simulink model "hnn_without_bias_3_neurons"  (R2024b)
settings: Solver=VariableStepAuto  StartTime=0.0  StopTime=10.0  RelTol=1e-3
settings Model: Creator=merlin  LastModifiedBy=merlin

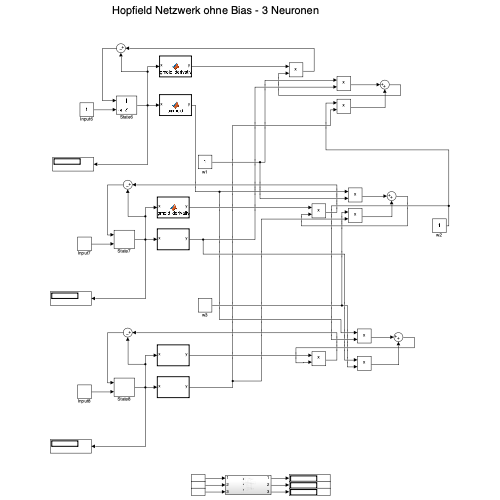
[thumbnail: Simulink's stored preview of the top-level diagram]
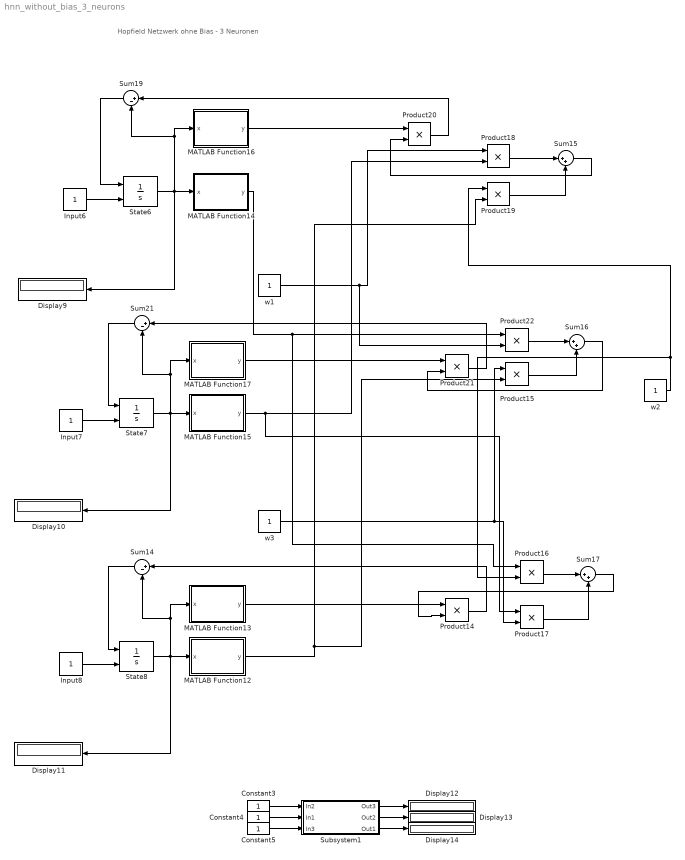
== system hnn_without_bias_3_neurons ==
  note: Hopfield Netzwerk ohne Bias - 3 Neuronen
  Constant3 : Constant
  Constant4 : Constant
  Constant5 : Constant
  Display{9..14} (6 alike) : Display
  Input6 : Constant
  Input7 : Constant
  Input8 : Constant
  MATLAB Function12 : MATLAB Function  TreatAsAtomicUnit=on
  MATLAB Function13 : MATLAB Function  TreatAsAtomicUnit=on
  MATLAB Function14 : MATLAB Function  TreatAsAtomicUnit=on
  MATLAB Function15 : MATLAB Function  TreatAsAtomicUnit=on
  MATLAB Function16 : MATLAB Function  TreatAsAtomicUnit=on
  MATLAB Function17 : MATLAB Function  TreatAsAtomicUnit=on
  Product{14..22} (9 alike) : Product
  State6 : Integrator  InitialConditionSource=external
  State7 : Integrator  InitialConditionSource=external
  State8 : Integrator  InitialConditionSource=external
  Subsystem1 : Subsystem
  Sum14 : Sum  Inputs=|+-
  Sum15 : Sum  Inputs=|++
  Sum16 : Sum  Inputs=|++
  Sum17 : Sum  Inputs=|++
  Sum19 : Sum  Inputs=|+-
  Sum21 : Sum  Inputs=|+-
  w1 : Constant
  w2 : Constant
  w3 : Constant
  wires:
  Sum14/1 -> State8/1
  Sum21/1 -> State7/1
  Sum17/1 -> Product14/2
  Product22/1 -> Sum16/1
  Input7/1 -> State7/2
  State7/1 -> Display10/1, Sum21/2, MATLAB Function17/1(x), MATLAB Function15/1(x)
  Product20/1 -> Sum19/1
  w3/1 -> Product17/2, Product15/1
  MATLAB Function16/1(y) -> Product20/1
  State6/1 -> Display9/1, Sum19/2, MATLAB Function16/1(x), MATLAB Function14/1(x)
  MATLAB Function12/1(y) -> Product15/2, Product19/2
  Subsystem1/2(Out2) -> Display13/1
  w2/1 -> Product16/2, Product19/1
  MATLAB Function17/1(y) -> Product21/1
  Input8/1 -> State8/2
  Sum19/1 -> State6/1
  Constant5/1 -> Subsystem1/3(In3)
  Constant4/1 -> Subsystem1/2(In1)
  Product15/1 -> Sum16/2
  MATLAB Function15/1(y) -> Product17/1, Product18/2
  Product14/1 -> Sum14/1
  Subsystem1/1(Out3) -> Display12/1
  Input6/1 -> State6/2
  State8/1 -> Display11/1, Sum14/2, MATLAB Function13/1(x), MATLAB Function12/1(x)
  w1/1 -> Product22/2, Product18/1
  Constant3/1 -> Subsystem1/1(In2)
  MATLAB Function14/1(y) -> Product16/1, Product22/1
  Product19/1 -> Sum15/2
  Product17/1 -> Sum17/2
  Sum15/1 -> Product20/2
  Product16/1 -> Sum17/1
  Product18/1 -> Sum15/1
  MATLAB Function13/1(y) -> Product14/1
  Sum16/1 -> Product21/2
  Subsystem1/3(Out1) -> Display14/1
  Product21/1 -> Sum21/1

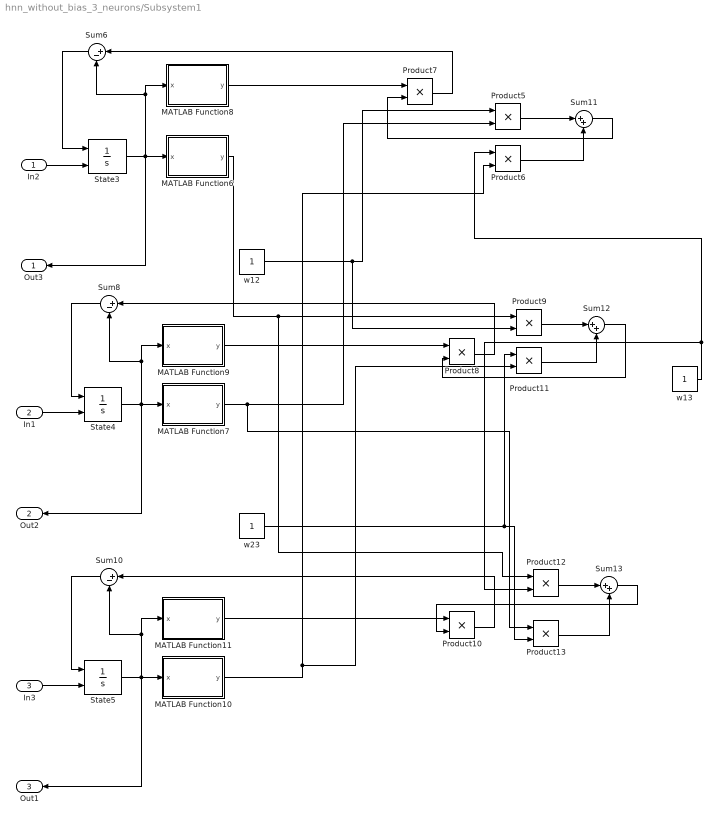
== system hnn_without_bias_3_neurons/Subsystem1 ==
  In2 : Inport
  In1 : Inport  Port=2
  In3 : Inport  Port=3
  MATLAB Function10 : MATLAB Function  TreatAsAtomicUnit=on
  MATLAB Function11 : MATLAB Function  TreatAsAtomicUnit=on
  MATLAB Function6 : MATLAB Function  TreatAsAtomicUnit=on
  MATLAB Function7 : MATLAB Function  TreatAsAtomicUnit=on
  MATLAB Function8 : MATLAB Function  TreatAsAtomicUnit=on
  MATLAB Function9 : MATLAB Function  TreatAsAtomicUnit=on
  Product{5..13} (9 alike) : Product
  State3 : Integrator  InitialConditionSource=external
  State4 : Integrator  InitialConditionSource=external
  State5 : Integrator  InitialConditionSource=external
  Sum10 : Sum  Inputs=|+-
  Sum11 : Sum  Inputs=|++
  Sum12 : Sum  Inputs=|++
  Sum13 : Sum  Inputs=|++
  Sum6 : Sum  Inputs=|+-
  Sum8 : Sum  Inputs=|+-
  w12 : Constant
  w13 : Constant
  w23 : Constant
  Out3 : Outport
  Out2 : Outport  Port=2
  Out1 : Outport  Port=3
  wires:
  Product9/1 -> Sum12/1
  Product13/1 -> Sum13/2
  Sum11/1 -> Product7/2
  Sum10/1 -> State5/1
  MATLAB Function7/1(y) -> Product13/1, Product5/2
  MATLAB Function9/1(y) -> Product8/1
  Product5/1 -> Sum11/1
  w12/1 -> Product9/2, Product5/1
  State5/1 -> Out1/1, Sum10/2, MATLAB Function11/1(x), MATLAB Function10/1(x)
  MATLAB Function8/1(y) -> Product7/1
  MATLAB Function11/1(y) -> Product10/1
  Sum13/1 -> Product10/2
  MATLAB Function6/1(y) -> Product12/1, Product9/1
  Product12/1 -> Sum13/1
  MATLAB Function10/1(y) -> Product11/2, Product6/2
  State4/1 -> Out2/1, Sum8/2, MATLAB Function9/1(x), MATLAB Function7/1(x)
  Sum8/1 -> State4/1
  Product8/1 -> Sum8/1
  State3/1 -> Out3/1, Sum6/2, MATLAB Function8/1(x), MATLAB Function6/1(x)
  Sum6/1 -> State3/1
  Product7/1 -> Sum6/1
  Product6/1 -> Sum11/2
  In1/1 -> State4/2
  Sum12/1 -> Product8/2
  In3/1 -> State5/2
  w23/1 -> Product13/2, Product11/1
  Product11/1 -> Sum12/2
  Product10/1 -> Sum10/1
  w13/1 -> Product12/2, Product6/1
  In2/1 -> State3/2

== matlab function hnn_without_bias_3_neurons/MATLAB Function13 ==
  data: x input; y output
function y = sigmoid_derivative(x)
sigmoid = 1 ./ (1 + exp(-x));
y = sigmoid .* (1 - sigmoid);
end

== matlab function hnn_without_bias_3_neurons/MATLAB Function14 ==
  data: x input; y output
function y = sigmoid(x)
y = 1 ./ (1 + exp(-x));
end

== matlab function hnn_without_bias_3_neurons/MATLAB Function15 ==
  data: x input; y output
function y = sigmoid(x)
y = 1 ./ (1 + exp(-x));
end

== matlab function hnn_without_bias_3_neurons/MATLAB Function16 ==
  data: x input; y output
function y = sigmoid_derivative(x)
sigmoid = 1 ./ (1 + exp(-x));
y = sigmoid .* (1 - sigmoid);
end

== matlab function hnn_without_bias_3_neurons/MATLAB Function17 ==
  data: x input; y output
function y = sigmoid_derivative(x)
sigmoid = 1 ./ (1 + exp(-x));
y = sigmoid .* (1 - sigmoid);
end

== matlab function hnn_without_bias_3_neurons/Subsystem1/MATLAB Function10 ==
  data: x input; y output
function y = sigmoid(x)
y = 1 ./ (1 + exp(-x));
end

== matlab function hnn_without_bias_3_neurons/Subsystem1/MATLAB Function11 ==
  data: x input; y output
function y = sigmoid_derivative(x)
sigmoid = 1 ./ (1 + exp(-x));
y = sigmoid .* (1 - sigmoid);
end

== matlab function hnn_without_bias_3_neurons/Subsystem1/MATLAB Function6 ==
  data: x input; y output
function y = sigmoid(x)
y = 1 ./ (1 + exp(-x));
end

== matlab function hnn_without_bias_3_neurons/MATLAB Function12 ==
  data: x input; y output
function y = sigmoid(x)
y = 1 ./ (1 + exp(-x));
end

== matlab function hnn_without_bias_3_neurons/Subsystem1/MATLAB Function7 ==
  data: x input; y output
function y = sigmoid(x)
y = 1 ./ (1 + exp(-x));
end

== matlab function hnn_without_bias_3_neurons/Subsystem1/MATLAB Function8 ==
  data: x input; y output
function y = sigmoid_derivative(x)
sigmoid = 1 ./ (1 + exp(-x));
y = sigmoid .* (1 - sigmoid);
end

== matlab function hnn_without_bias_3_neurons/Subsystem1/MATLAB Function9 ==
  data: x input; y output
function y = sigmoid_derivative(x)
sigmoid = 1 ./ (1 + exp(-x));
y = sigmoid .* (1 - sigmoid);
end
